simulink model "samolet"  (Simulink 7.3)
settings: Solver=ode45  StartTime=0.0  StopTime=10  RelTol=1e-3
undefined symbols (not defined in the file or in its folder): DiscIntNeverNeededParam
settings Model: Creator=Sainquake Notebook  LastModifiedBy=Sainquake Notebook

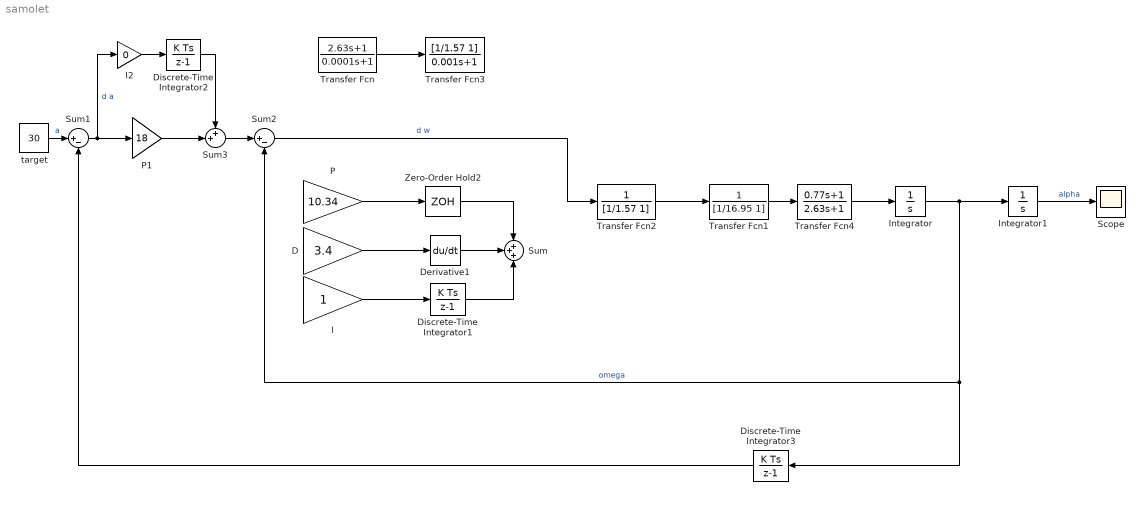
== system samolet ==
  D : Gain  Gain=3.4  ParameterDataType=fixdt(1, 16)  ParameterScaling=2^0  OutDataType=fixdt(1, 16)  OutScaling=2^0
  Derivative1 : Derivative
  Discrete-Time Integrator1 : DiscreteIntegrator  SampleTime=1/200  OutDataType=fixdt(1, 16)  OutScaling=2^0  ICPrevOutput=DiscIntNeverNeededParam  ICPrevScaledInput=DiscIntNeverNeededParam
  Discrete-Time Integrator2 : DiscreteIntegrator  SampleTime=1/200  OutDataType=fixdt(1, 16)  OutScaling=2^0  ICPrevOutput=DiscIntNeverNeededParam  ICPrevScaledInput=DiscIntNeverNeededParam
  Discrete-Time Integrator3 : DiscreteIntegrator  SampleTime=1/200  OutDataType=fixdt(1, 16)  OutScaling=2^0  ICPrevOutput=DiscIntNeverNeededParam  ICPrevScaledInput=DiscIntNeverNeededParam
  I : Gain  ParameterDataType=fixdt(1, 16)  ParameterScaling=2^0  OutDataType=fixdt(1, 16)  OutScaling=2^0
  I2 : Gain  Gain=0  ParameterDataType=fixdt(1, 16)  ParameterScaling=2^0  OutDataType=fixdt(1, 16)  OutScaling=2^0
  Integrator : Integrator
  Integrator1 : Integrator
  P : Gain  Gain=10.34  ParameterDataType=fixdt(1, 16)  ParameterScaling=2^0  OutDataType=fixdt(1, 16)  OutScaling=2^0
  P1 : Gain  Gain=18  ParameterDataType=fixdt(1, 16)  ParameterScaling=2^0  OutDataType=fixdt(1, 16)  OutScaling=2^0
  Scope : Scope
      settings: YMin=-2.25e+006  YMax=750000  MaxDataPoints=500000
  Sum : Sum  Inputs=+++  OutDataType=fixdt(1, 16)  OutScaling=2^0
  Sum1 : Sum  Inputs=|+-  OutDataType=fixdt(1, 16)  OutScaling=2^0
  Sum2 : Sum  Inputs=|+-  OutDataType=fixdt(1, 16)  OutScaling=2^0
  Sum3 : Sum  Inputs=++|  OutDataType=fixdt(1, 16)  OutScaling=2^0
  Transfer Fcn : TransferFcn  Numerator=[2.63 1]  Denominator=[0.0001 1]
  Transfer Fcn1 : TransferFcn  Numerator=1  Denominator=[1/16.95 1]
  Transfer Fcn2 : TransferFcn  Numerator=1  Denominator=[1/1.57 1]
  Transfer Fcn3 : TransferFcn  Numerator=[1/1.57 1]  Denominator=[0.001 1]
  Transfer Fcn4 : TransferFcn  Numerator=[0.77 1]  Denominator=[2.63 1]
  Zero-Order Hold2 : ZeroOrderHold  SampleTime=1/200
  target : Constant  Value=30  OutDataType=fixdt(1, 16)  OutScaling=2^0
  wires:
  D/1 -> Derivative1/1
  I/1 -> Discrete-Time Integrator1/1
  Discrete-Time Integrator1/1 -> Sum/3
  Integrator/1 -> Integrator1/1, Discrete-Time Integrator3/1, Sum2/2  "omega"
  Integrator1/1 -> Scope/1  "alpha"
  Transfer Fcn2/1 -> Transfer Fcn1/1
  Transfer Fcn1/1 -> Transfer Fcn4/1
  Transfer Fcn4/1 -> Integrator/1
  Derivative1/1 -> Sum/2
  Transfer Fcn/1 -> Transfer Fcn3/1
  P/1 -> Zero-Order Hold2/1
  target/1 -> Sum1/1  "a"
  Discrete-Time Integrator3/1 -> Sum1/2
  Zero-Order Hold2/1 -> Sum/1
  Sum3/1 -> Sum2/1
  P1/1 -> Sum3/2
  Sum1/1 -> P1/1, I2/1  "d a"
  Discrete-Time Integrator2/1 -> Sum3/1
  I2/1 -> Discrete-Time Integrator2/1
  Sum2/1 -> Transfer Fcn2/1  "d w"
